simulink model "simulacaoSimulink"  (R2016a)
settings: Solver=VariableStepAuto  SolverMode=SingleTasking  StartTime=0.0  StopTime=500  RelTol=1e-3
settings Model: Creator=jhull  LastModifiedBy=jhull
settings DataIOCC: ReturnWorkspaceOutputs=on
settings DebuggingCC: SFUnexpectedBacktrackingDiag=error  SFNoUnconditionalDefaultTransitionDiag=error
settings SFSimCC: SimUseLocalCustomCode=on
settings RTWCC: RTWUseLocalCustomCode=on
settings GRTTargetCC: TargetLangStandard=C99 (ISO)
settings ConfigComp: CovMetricSettings=dwe  CovSaveCumulativeToWorkspaceVar=off  CovSaveSingleToWorkspaceVar=off  CovExternalEMLEnable=on

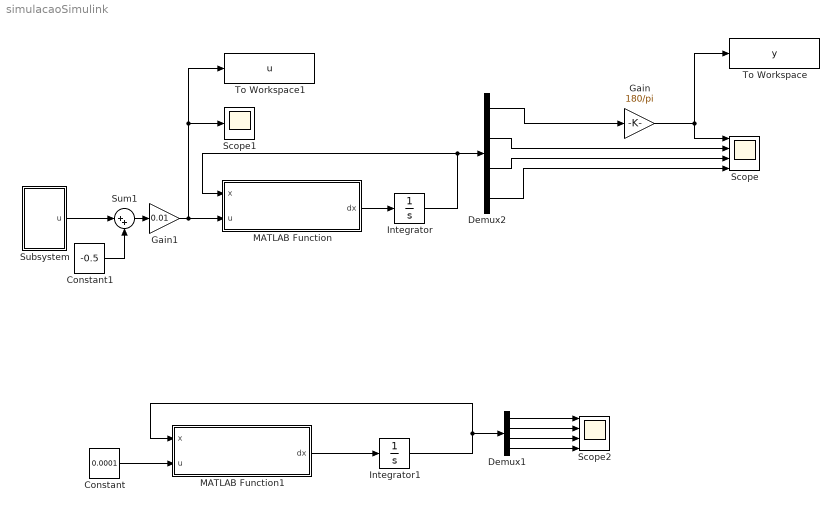
== system simulacaoSimulink ==
  Constant : Constant  Value=0.0001
  Constant1 : Constant  Value=-0.5
  Demux1 : Demux
  Demux2 : Demux
  Gain : Gain  Gain=180/pi
  Gain1 : Gain  Gain=0.01
  Integrator : Integrator  InitialCondition=[pi;0;0;0]
  Integrator1 : Integrator  InitialCondition=[0;0;0;0]
  MATLAB Function : MATLAB Function  TreatAsAtomicUnit=on
  MATLAB Function1 : MATLAB Function  TreatAsAtomicUnit=on
  Scope : Scope  NumInputPorts=4
  Scope1 : Scope
  Scope2 : Scope  NumInputPorts=4
  Subsystem : Subsystem
  Sum1 : Sum  Inputs=|++
  To Workspace : ToWorkspace  VariableName=y  SaveFormat=Timeseries  SampleTime=-1
  To Workspace1 : ToWorkspace  VariableName=u  SaveFormat=Timeseries  SampleTime=-1
  wires:
  Demux2/1 -> Gain/1
  Demux2/2 -> Scope/2
  Demux2/3 -> Scope/3
  Demux2/4 -> Scope/4
  Integrator/1 -> MATLAB Function/1(x), Demux2/1
  MATLAB Function/1(dx) -> Integrator/1
  Constant/1 -> MATLAB Function1/2(u)
  MATLAB Function1/1(dx) -> Integrator1/1
  Demux1/3 -> Scope2/3
  Demux1/1 -> Scope2/1
  Demux1/4 -> Scope2/4
  Integrator1/1 -> MATLAB Function1/1(x), Demux1/1
  Demux1/2 -> Scope2/2
  Constant1/1 -> Sum1/2
  Subsystem/1(u) -> Sum1/1
  Gain/1 -> To Workspace/1, Scope/1
  Sum1/1 -> Gain1/1
  Gain1/1 -> To Workspace1/1, Scope1/1, MATLAB Function/2(u)

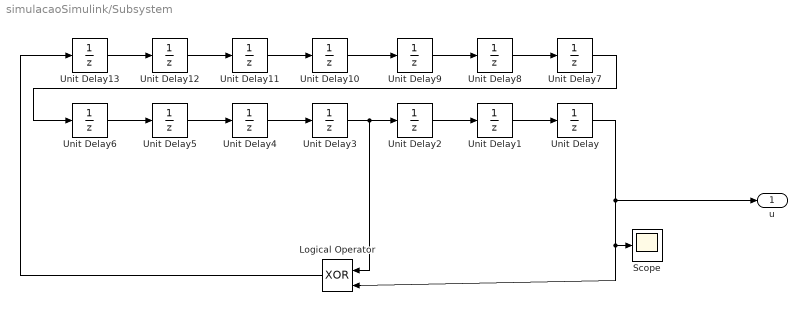
== system simulacaoSimulink/Subsystem ==
  Logical Operator : Logic  Operator=XOR  IconShape=distinctive  AllPortsSameDT=off  OutDataTypeStr=boolean
  Scope : Scope
  Unit Delay{,1..13} (14 alike) : UnitDelay  InitialCondition=1  HasFrameUpgradeWarning=on
  u : Outport
  wires:
  Unit Delay3/1 -> Logical Operator/1, Unit Delay2/1
  Unit Delay/1 -> u/1, Logical Operator/2, Scope/1
  Unit Delay6/1 -> Unit Delay5/1
  Unit Delay5/1 -> Unit Delay4/1
  Unit Delay1/1 -> Unit Delay/1
  Unit Delay2/1 -> Unit Delay1/1
  Unit Delay4/1 -> Unit Delay3/1
  Unit Delay12/1 -> Unit Delay11/1
  Unit Delay11/1 -> Unit Delay10/1
  Unit Delay10/1 -> Unit Delay9/1
  Unit Delay9/1 -> Unit Delay8/1
  Unit Delay13/1 -> Unit Delay12/1
  Unit Delay8/1 -> Unit Delay7/1
  Logical Operator/1 -> Unit Delay13/1
  Unit Delay7/1 -> Unit Delay6/1

== matlab function simulacaoSimulink/MATLAB Function1 ==
  data: x input; u input; dx output

function dx = PenduloInvertido(x, u)
%O que deu mais certo 
    % Parâmetros do sistema
    m = 0.1;    % Massa pendurada
    M = 1;      % Massa do carro
    l = 0.5;    % Comprimento do pêndulo
    b = 0.1;    % Coeficiente de amortecimento
    g = 9.8;    % Aceleração devida à gravidade
    J = (m*l^2)/3; % Momento de inércia do pêndulo em relação ao eixo vertical

    % Equações diferenciais
    dx1 = x(2);
    dx2 = (1/(M+m)) * (m*g*l*sin(x(1)) - b*x(2) + l*cos(x(1))*u);
    dx3 = x(4);
    dx4 = (1/((M+m)*l^2)) * (m*l*cos(x(1))*x(2)^2 - (M+m)*g*l*sin(x(1)) - b*l*x(4) + l*u*cos(x(1)));
    
    % Vetor de saída
    dx = [dx1; dx2; dx3; dx4];
end

== matlab function simulacaoSimulink/MATLAB Function ==
  data: x input; u input; dx output
function dx = PenduloInvertido(x, u)
    % Parâmetros do sistema
    m = 0.1;    % Massa pendurada
    M = 1;      % Massa do carro
    l = 0.5;    % Comprimento do pêndulo
    b = 0.1;    % Coeficiente de amortecimento
    g = 9.8;    % Aceleração devida à gravidade

    % Equações diferenciais
    dx1 = x(2);
    dx2 = (1/(M+m)) * (m*g*l*sin(x(1)) - b*x(2) + l*cos(x(1))*u);
    dx3 = x(4);
    dx4 = (1/((M+m)*l^2)) * (m*l*cos(x(1))*x(2)^2 - (M+m)*g*l*sin(x(1)) - b*l*x(4) + l*u*cos(x(1)));
    
    % Vetor de saída
    dx = [dx1; dx2; dx3; dx4];
end
